simulink model "single-phase full- bridge-controlled rectifier"  (R2022a)
settings: Solver=VariableStepAuto  StartTime=0.0  StopTime=0.1  RelTol=1e-3
libraries: spsDiodeLib x4, spsCurrentMeasurementLib x3, spsSeriesRLCBranchLib x3, spsVoltageMeasurementLib x2, spsACVoltageSourceLib x1, spspowerguiLib x1
settings Model: Creator=Joy  LastModifiedBy=Joy
settings SolverCC: AlgebraicLoopSolver=TrustRegion

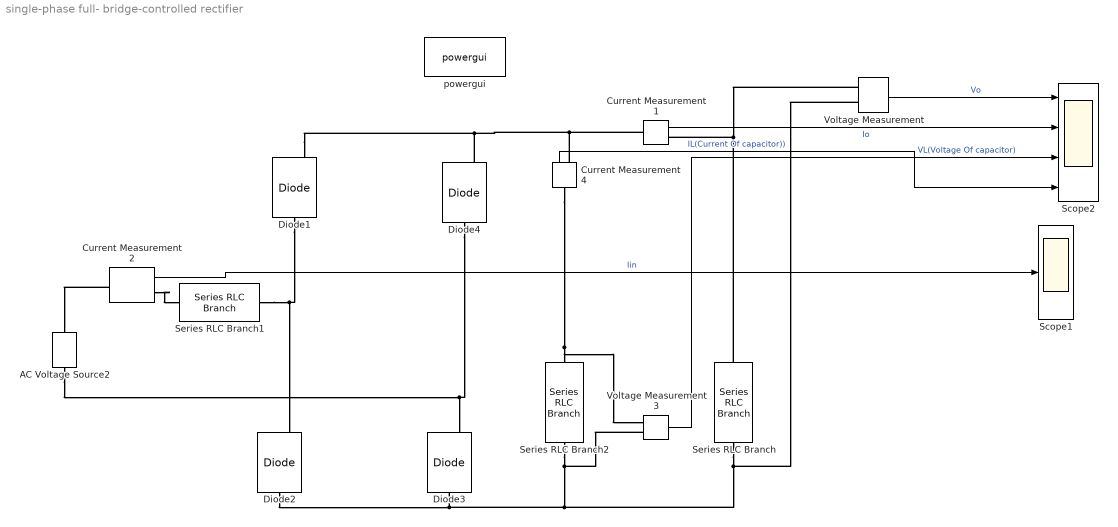
== system single-phase full- bridge-controlled rectifier ==
  AC Voltage Source2 : spsACVoltageSourceLib/AC Voltage Source  Amplitude=325.26  Phase=0  Frequency=100  SampleTime=0  Measurements=Voltage  BusType=swing  Pref=10e3  Qref=0  Qmin=-inf  Qmax=+inf
  Current Measurement1 : spsCurrentMeasurementLib/Current Measurement  PhasorSimulation=off  OutputType=Complex  PSBequivalent=0
  Current Measurement2 : spsCurrentMeasurementLib/Current Measurement  PhasorSimulation=off  OutputType=Complex  PSBequivalent=0
  Current Measurement4 : spsCurrentMeasurementLib/Current Measurement  PhasorSimulation=off  OutputType=Complex  PSBequivalent=0
  Diode{1..4} (4 alike) : spsDiodeLib/Diode  Ron=0.001  Lon=0  Vf=0.8  IC=0  UseSnubber=0  Rs=500  Cs=250e-9  Measurements=on
  Scope1 : Scope
  Scope2 : Scope  NumInputPorts=4
  Series RLC Branch : spsSeriesRLCBranchLib/Series RLC Branch  LConnTagsString=__new0  RConnTagsString=__new0  BranchType=R  Resistance=20  Inductance=1e-3  SetiL0=off  InitialCurrent=0  Capacitance=1e-6  Setx0=off  InitialVoltage=0  Measurements=None
  Series RLC Branch1 : spsSeriesRLCBranchLib/Series RLC Branch  LConnTagsString=__new0  RConnTagsString=__new0  BranchType=L  Resistance=1  Inductance=2e-3  SetiL0=off  InitialCurrent=0  Capacitance=1e-6  Setx0=off  InitialVoltage=0  Measurements=None
  Series RLC Branch2 : spsSeriesRLCBranchLib/Series RLC Branch  LConnTagsString=__new0  RConnTagsString=__new0  BranchType=C  Resistance=1  Inductance=1e-3  SetiL0=off  InitialCurrent=0  Capacitance=1e-6  Setx0=off  InitialVoltage=0  Measurements=None
  Voltage Measurement : spsVoltageMeasurementLib/Voltage Measurement  PhasorSimulation=off  OutputType=Complex  PSBequivalent=0
  Voltage Measurement3 : spsVoltageMeasurementLib/Voltage Measurement  PhasorSimulation=off  OutputType=Complex  PSBequivalent=0
  powergui : spspowerguiLib/powergui  Priority=1  SimulationMode=Continuous  SampleTime=50e-6  frequency=60  Iterations=50  frequencyindice=0  Pbase=100e6  ErrMax=1e-4  UnitsV=kV  UnitsW=MW  buscounter=0  FunctionMessages=off  echomessages=off  EnableUseOfTLC=off  CurrentSourceSwitches=off  DisableSnubberDevices=off  DisableRonSwitches=off  DisableVfSwitches=off  DisplayEquations=off  AutomaticDiscreteSolvers=off  SolverType=Tustin/Backward Euler (TBE)  Interpol=off  ExternalGateDelay=off  methode=off  Ts=100  x0status=blocks  SPID=on  SwTol=0  HookPort=off  NonlinearTolerance=1e-4  nMaxIteration=100  ContinueOnMaxIteration=off  RestoreLinks=warning  ResistiveCurrentMeasurement=off  Frange=[0:2:500]  Ylog=off  Xlog=on  ShowGrid=off  save=off  variable=ZData  structure=0  ZoomFFT=off  StartTime=0.0  cycles=1  DisplayStyle=1  fundamental=60  FreqAxis=off  MaxFrequency=1000  frequencyindicesteady=1  RmsSteady=1  display=off
  wires:
  Voltage Measurement/1 -> Scope2/1  "Vo"
  Current Measurement1/1 -> Scope2/2  "Io"
  Voltage Measurement3/1 -> Scope2/3  "VL(Voltage Of capacitor)"
  Current Measurement4/1 -> Scope2/4  "IL(Current Of capacitor))"
  Current Measurement2/1 -> Scope1/1  "Iin"
  connections:
  Diode1/RConn1 -- Current Measurement4/RConn1 -- Current Measurement1/LConn1 -- Diode4/RConn1
  Series RLC Branch1/RConn1 -- Diode1/LConn1 -- Diode2/RConn1
  Diode2/LConn1 -- Voltage Measurement3/LConn2 -- Series RLC Branch2/RConn1 -- Voltage Measurement/LConn2 -- Series RLC Branch/RConn1 -- Diode3/LConn1
  AC Voltage Source2/LConn1 -- Diode4/LConn1 -- Diode3/RConn1
  Series RLC Branch/LConn1 -- Current Measurement1/RConn1 -- Voltage Measurement/LConn1
  Series RLC Branch2/LConn1 -- Voltage Measurement3/LConn1 -- Current Measurement4/LConn1
  Current Measurement2/RConn1 -- Series RLC Branch1/LConn1
  Current Measurement2/LConn1 -- AC Voltage Source2/RConn1
